simulink model "case14"  (R2018b)
settings: Solver=VariableStepAuto  StartTime=0.0  StopTime=10.0  RelTol=1e-3
(part 2 of 2)

== matlab function case14/MATLAB Function3 ==
  data: y output
function y = fcn()

 u=[0,1,1,1,1,0,1,1,1,1,0,0,1,0,1,0,1,0,1,0,0,1,0,1,1,1,0,1,1,0,0,1,1,0,0,0,1,1,0,0,0,0,1,1,0,0,1,0,1,1,1,0,0,1,1,1,1,0,0,0,0,1,1,1,1,1,0,0,0,1,0,1,1,1,1,1,0,0,0,0,0,1,0,1,1,1,1,0,0,0,0,0,1,1,0,1,1,0,1,0,1,1,0,0,0,0,1,1,1,0,1,1,1,1,0,0,0,0,0,0,0,1,1,0,1,0,1,1,1,1,1,0,0,0,0,0,0,0,1,1,0,0,1,1,1,1,1,1,1,0,1,1,0,0,0,0,0,0,0,1,0,1,1,1,0,1,1,0,1,1,1,0,1,1,0,1,0,0,0,0,0,1,0,1,1,0,1,1,0,1,1,0,1,1,0,1,1,0,0,1,1,0,1,0,0,1,0,1,0,1,0,0,1,1,1,0,1,1,0,1,1,1,1,0,1,1,1,1,0,1,0,0,0,1,0,1,0,0,0,1,0,0,1,1,1,0,0,1,1,1,0,1,1,0,1,1,1,1,1,1,1,0,0,1,0,0,0,0,0,1,0,0,0,0,0,0,1,0,1,1,0,0,0,1,1,1,1,0,1,1,1,0,1,0,1,1,1,0,0,0,1,1,1,1,0,0,0,1,0,0,0,1,0,0,0,0,0,1,1,1,0,1,1,1,1,0,1,0,0,0,1,0,1,1,0,1,1,1,1,1,1,0,0,1,1,0,1,0,0,0,1,0,0,0,0,0,0,0,0,1,0,1,1,1,0,0,1,1,1,0,0,1,1,1,1,0,0,1,1,0,1,1,0,0,1,1,1,1,0,0,1,0,1,0,0,1,0,1,1,0,1,1,0,0,1,0,0,0,0,1,1,0,0,0,1,0,0,1,1,1,0,1,0,0,1,0,1,1,1,1,0,1,1,1,1,1,0,0,1,0,1,1,1,1,1,1,0,0,1,0,1,1,1,1,1,1,0,1,1,0,0,1,0,1,0,0,1,1,0,0,1,0,0,0,0,0,0,1,1,1,0,0,0,1,1,1,1,1,1,1,0,0,0,1,1,1,1,1,1,1,0,0,1,1,1,0,0,1,1,1,1,1,1,0,1,1,1,1,1,1,1,1,0,1,0,1,1,0,0,1,0,0,0,1,0,0,0,0,1,0,0,0,0,1,0,1,0,0,0,1,0,1,1,0,0,0,1,1,1,0,0,1,0,1,0,0,1,1,1,0,1,1,1,0,0,1,1,1,1,1,1,1,0,0,1,1,0,1,1,0,1,0,1,1,0,1,0,1,0,0,1,1,1,0,1,0,1,0,0,0,0,1,0,1,1,1,0,1,0,0,0,1,1,0,0,1,0,1,0,0,0,0,0,0,1,0,1,0,1,1,0,0,1,1,1,0,1,1,1,1,0,1,1,1,0,1,0,1,0,1,1,0,0,1,1,1,1,0,0,0,1,0,1,1,1,1,1,0,1,0,1,1,0,1,0,1,1,1,1,0,0,0,1,0,0,0,0,1,0,1,1,0,0,0,0,1,0,1,0,1,0,0,0,1,0,0,0,1,1,1,0,0,1,0,1,0,1,1,0,1,0,0,1,0,1,0,1,1,0,0,0,1,1,0,1,1,1,1,1,1,0,0,0,1,1,0,1,0,0,0,1,1,1,0,0,1,0,1,1,1,1,1,1,0,1,1,0,1,0,1,1,0,0,0,1,1,0,0,0,1,1,1,0,0,1,0,1,0,0,1,1,0,1,0,0,0,0,1,1,0,0,1,0,0,0,0,0,0,1,0,1,0,0,1,0,0,0,1,1,1,0,0,0,0,1,1,1,1,1,1,0,1,1,0,0,0,0,1,1,1,0,1,1,0,1,1,1,1,1,1,0,0,1,0,1,0,1,1,1,1,1,1,0,0,0,0,1,1,0,0,1,0,1,1,1,1,1,1,1,1,1,0,0,1,0,1,1,0,0,0,1,0,1,1,1,0,1,0,1,1,1,1,0,0,1,0,1,0,0,0,0,1,1,0,0,1,1,0,0,1,0,0,1,1,1,0,0,0,0,0,1,0,0,0,0,0,0,1,0,0,0,1,0,0,1,1,1,1,1,0,0,1,0,1,0,0,1,0,1,1,1,0,1,1,1,0,1,1,1,1,0,0,0,0,0,1,1,0,1,1,1,0,1,0,1,0,1,0,1,1,0,1,0,1,1,1,1,0,1,0,0,1,0,1,1,1,1,1,1,0,1,0,1,0,1,0,0,1,1,1,1,1,1,0,1,0,1,0,1,1,1,0,1,0,0,0,1,0,0,1,1,1,1,0,0,1,0,1,1,0,0,0,0,1,0,0,1,1,0,0,0,0,0,0,0,1,1,1,0,0,0,0,0,1,0,0,1,0,0,1,1,0,0,0,0,0,0,0,1,0,0,1,1,0,1,0,0,0,0,0,0,0,1,1,1,1,1,0,0,1,0,1,1,1,0,0,1,1,0,0,0,1,1,1,1,0,1,0,0,1,1,1,1,1,1,0,0,1,0,0,1,0,1,0,1,1,1,1,1,0,1,1,1,1,0,0,0,0,1,0,1,0,0,0,1,0,1,0,0,0,1,0,0,1,1,1,1,0,0,1,1,1,0,1,1,0,0,0,0,1,1,0,1,1,1,1,0,0,1,0,0,1,1,0,0,0,0,0,0,1,0,0,1,1,0,1,1,1,1,1,1,1,0,0,1,0,0,1,0,0,0,0,1,0,1,0,0,0,0,1,1,1,0,0,1,0,0,1,0,0,0,1,0,1,0,1,0,1,1,0,0,0,1,1,0,0,1,0,1,1,0,1,0,0,1,0,1,1,1,0,0,0,1,1,1,0,1,0,1,1,0,0,1,0,1,1,1,1,0,1,1,0,0,0,1,0,0,0,1,0,1,0,0,1,0,1,1,0,1,1,1,0,1,1,0,1,0,0,0,1,1,0,0,1,1,0,1,0,1,0,1,1,1,1,0,1,1,0,0,1,1,1,1,1,0,1,1,1,0,1,1,1,1,1,1,1,1,0,0,0,0,0,0,1,1,1,0,0,0,1,0,0,0,1,1,0,0,0,1,1,1,1,0,1,0,1,0,0,0,1,1,0,0,0,1,0,0,1,1,0,0,0,0,1,0,0,1,1,0,0,0,1,0,0,1,1,1,1,1,0,0,1,0,0,1,0,0,1,1,1,0,1,1,1,1,1,0,0,1,1,0,1,0,1,1,1,0,1,1,0,0,1,1,0,1,0,0,0,0,1,0,1,1,0,1,1,0,1,1,1,1,1,1,0,1,1,1,1,1,0,0,1,0,0,0,0,1,1,1,1,0,0,1,1,0,0,0,0,0,1,1,1,1,1,1,1,0,1,0,0,1,1,0,1,1,0,1,0,1,0,1,0,1,1,1,1,0,1,1,0,1,1,0,1,1,0,0,1,1,0,1,0,0,1,0,1,0,1,1,1,1,1,0,0,0,1,0,0,1,0,1,0,1,1,0,0,0,1,1,1,0,1,1,0,0,0,0,1,1,1,1,0,0,1,1,0,0,0,0,1,0,0,0,0,1,0,1,0,0,0,0,0,1,0,0,1,0,0,0,1,0,1,0,1,0,1,1,0,0,1,1,0,0,1,0,1,1,1,0,1,0,0,0,1,1,1,1,1,1,0,0,0,0,1,0,0,0,0,1,0,1,1,1,1,1,0,1,0,1,1,0,1,1,1,1,0,0,0,0,1,0,1,0,0,1,0,1,1,1,1,0,1,1,1,1,1,0,0,1,1,1,1,1,1,1,0,1,0,1,0,0,0,0,0,1,1,0,1,1,1,0,1,1,1,1,1,1,1,1,0,1,0,1,1,0,1,0,1,0,0,0,1,1,1,1,1,0,1,0,0,1,1,0,0,1,1,1,0,1,0,1,0,1,0,1,1,1,0,1,1,1,1,0,0,0,1,1,1,0,1,1,1,1,0,0,0,0,0,0,1,1,0,0,1,1,0,1,0,1,0,0,1,1,1,0,0,1,0,1,0,1,0,1,0,0,1,0,0,1,0,0,0,1,1,0,0,0,1,0,1,0,1,1,1,1,1,0,1,0,1,1,1,1,1,0,0,0,0,1,0,0,0,0,1,1,0,1,1,1,0,0,1,0,1,0,1,0,1,0,1,1,1,0,1,0,0,0,0,0,0,0,1,0,0,1,1,0,0,0,0,0,1,1,0,0,0,0,1,1,1,1,0,1,0,1,1,1,1,0,0,0,0,1,0,0,0,1,1,0,1,0,1,1,1,0,0,1,1,1,0,1,1,0,1,1,1,1,1,1,1,0,0,1,1,1,1,1,1,1,1,0,1,0,0,0,1,0,0,0,1,1,1,1,0,0,0,1,1,1,0,1,1,0,0,1,0,0,1,1,1,0,0,1,1,0,1,1,0,1,0,0,0,1,0,0,0,1,0,1,0,1,1,1,0,0,1,1,1,0,1,0,0,1,1,0,1,1,0,1,0,1,0,1,0,1,1,1,0,0,1,1,1,0,1,1,0,0,0,1,1,0,0,0,0,1,1,1,0,1,0,1,1,1,0,1,1,0,0,1,0,0,1,1,0,0,1,1,0,1,0,1,1,0,0,1,0,0,0,0,0,0,1,1,0,0,0,0,1,1,1,1,1,1,0,1,0,0,1,0,0,1,0,0,1,1,1,1,0,0,0,0,1,0,0,0,1,1,1,0,1,0,0,1,0,1,0,0,1,0,1,0,1,0,1,0,0,0,0,0,1,1,1,1,1,1,0,0,1,0,0,0,1,0,0,0,0,1,1,0,0,0,1,1,0,0,0,0,1,1,0,1,1,0,0,0,1,0,1,0,0,0,0,0,0,0,1,1,0,0,0,0,1,1,1,1,0,0,1,1,1,0,1,0,0,0,0,0,0,0,1,0,0,0,1,1,0,1,1,1,0,1,0,1,1,0,1,0,1,1,0,0,1,1,0,1,1,1,1,0,0,0,0,1,0,1,0,0,1,0,1,0,1,1,1,1,0,1,0,1,0,0,0,1,0,0,0,0,0,1,1,1,1,1,1,1,0,1,0,1,0,0,1,0,0,1,1,0,1,0,0,1,1,0,0,1,0,0,1,1,1,1,0,1,1,1,0,1,0,0,0,1,1,1,1,1,1,1,1,0,1,0,1,0,1,0,0,1,1,0,0,1,0,0,0,0,1,0,0,1,0,0,1,1,0,0,1,0,1,0,1,1,0,0,0,0,1,1,1,1,0,1,1,1,1,0,1,0,1,1,0,1,0,1,1,0,0,1,0,1,1,0,0,0,0,0,0,0,1,1,0,1,1,0,0,1,1,1,0,1,0,1,0,0,0,0,0,1,1,0,1,0,1,1,1,1,0,0,0,0,0,0,0,0,1,0,0,0,1,1,0,0,1,0,0,1,0,1,0,0,0,1,0,1,1,1,1,1,0,1,0,1,1,1,0,0,0,0,1,1,1,0,0,0,1,1,0,0,1,0,0,0,1,0,1,1,0,0,1,1,1,0,0,0,0,0,0,0,0,1,0,1,0,1,1,0,1,0,0,1,0,0,1,0,1,1,0,0,1,0,0,0,0,1,1,0,1,1,1,0,0,1,1,0,1,1,0,1,0,0,1,0,1,0,1,1,0,1,1,0,0,0,1,1,1,0,0,1,0,1,0,0,1,1,0,0,1,0,0,1,1,0,1,1,1,1,0,1,1,0,1,0,1,0,0,1,0,1,0,1,0,0,0,1,0,0,0,1,1,1,1,0,1,0,1,1,0,0,1,1,1,1,1,1,1,1,0,0,0,1,0,1,0,0,1,0,0,0,1,1,0,0,1,0,0,0,1,1,0,0,1,1,0,0,0,0,0,1,0,0,1,1,1,1,0,0,1,1,0,1,0,1,1,0,1,1,0,1,1,0,1,1,1,0,0,0,1,0,1,1,1,1,0,0,1,0,1,1,1,1,1,0,0,1,1,0,1,1,0,0,0,1,1,1,0,1,1,1,0,0,1,1,1,1,0,0,0,0,0,1,1,1,0,1,0,1,0,1,1,0,0,1,0,1,1,1,1,0,0,1,0,1,1,1,1,1,0,1,1,1,0,1,0,1,1,0,0,0,0,0,0,0,0,0,1,0,1,1,0,1,0,1,0,0,1,0,1,0,1,1,1,0,0,0,1,0,0,1,1,1,1,0,0,0,0,0,1,1,0,1,1,1,0,1,1,0,0,1,1,0,1,1,0,0,1,0,0,0,0,1,0,1,0,0,0,0,1,0,0,1,0,0,1,0,0,1,0,1,0,0,1,0,1,0,0,0,1,1,0,0,0,0,0,1,1,1,0,0,1,0,0,0,0,1,1,0,1,0,0,1,0,1,1,1,0,1,0,1,0,0,1,0,0,1,1,0,0,0,1,1,1,0,0,0,0,1,0,1,1,1,1,0,0,1,1,1,0,1,1,1,0,1,0,0,0,0,1,1,0,1,1,0,1,1,0,0,0,1,1,1,0,1,1,0,1,1,0,1,1,0,1,0,0,1,0,1,1,0,1,1,0,0,0,0,1,0,1,0,0,1,0,0,0,1,1,1,0,0,1,1,1,1,0,0,0,1,0,1,0,1,0,1,1,1,1,1,0,0,1,1,1,1,0,1,0,1,1,1,1,0,0,0,1,1,1,0,0,0,0,0,1,0,0,1,0,1,1,1,1,1,1,0,0,0,0,1,1,1,0,0,0,0,1,0,1,0,1,0,0,1,1,1,1,1,1,1,1,1,1,1,0,1,1,0,1,1,0,0,0,0,0,1,0,1,0,0,0,1,0,1,0,0,1,1,0,0,0,1,0,0,0,1,1,0,0,1,0,1,1,1,0,1,1,0,1,1,1,1,0,0,0,1,1,1,0,0,0,1,0,1,0,0,0,0,0,1,1,1,1,0,0,1,1,0,0,0,0,1,0,0,0,1,1,0,1,1,0,1,1,1,1,1,0,1,0,0,1,0,1,0,1,1,0,0,1,0,1,1,1,0,0,1,1,0,0,1,1,1,0,0,1,0,1,0,1,1,1,1,0,1,0,0,0,1,0,1,1,0,1,0,1,0,1,0,0,1,0,1,1,1,1,1,1,0,0,0,1,1,0,1,1,0,0,0,0,0,0,0,0,1,0,0,1,0,1,0,1,0,1,1,1,0,1,1,1,0,0,0,0,0,1,0,1,0,0,1,0,0,1,0,1,1,0,0,1,0,0,0,0,1,1,0,0,1,0,0,0,1,1,0,1,1,0,1,0,0,0,0,0,1,0,1,0,0,0,0,0,1,0,0,1,1,0,1,0,1,0,0,0,1,0,0,1,0,1,0,1,1,0,1,0,1,0,1,0,1,0,1,1,0,1,0,0,0,0,0,0,1,0,0,1,0,1,0,0,0,1,1,0,0,1,1,0,1,1,1,1,1,1,1,1,0,0,1,1,0,1,1,1,1,0,0,1,1,1,1,0,1,0,1,1,0,0,0,1,0,0,0,0,1,0,0,1,1,0,0,1,0,0,1,0,0,0,1,1,1,1,1,0,1,1,0,1,1,0,1,0,1,0,1,1,1,0,0,1,0,0,1,1,1,0,1,0,1,1,1,0,1,0,1,1,0,0,1,0,0,0,1,0,0,0,0,1,0,1,0,1,0,0,1,1,1,1,0,0,1,1,1,1,1,0,0,0,1,1,1,1,1,0,1,1,1,1,1,1,1,1,1,0,0,1,1,1,0,1,1,0,1,0,0,1,1,0,0,1,1,0,0,0,0,0,0,0,1,1,1,1,1,0,1,0,1,0,0,0,1,1,0,0,0,0,1,1,1,1,0,0,0,0,1,0,1,0,1,0,0,0,1,0,0,0,1,1,0,0,1,0,0,1,1,1,1,0,1,0,0,1,1,1,1,1,1,0,1,1,0,0,0,1,0,1,1,0,1,1,1,1,0,1,1,1,1,1,1,1,1,0,0,1,0,0,0,0,0,1,0,0,0,1,1,0,1,1,0,0,0,1,1,0,1,1,0,0,1,0,0,1,1,0,0,1,0,0,1,1,1,1,1,0,0,1,0,1,1,1,0,0,1,1,0,0,1,1,0,0,1,0,0,1,0,1,1,0,0,1,0,1,1,1,0,1,0,1,0,0,1,1,1,0,0,1,0,1,0,1,1,1,0,1,1,0,0,1,1,0,1,0,1,1,1,0,1,0,0,1,1,1,0,1,1,0,1,1,1,1,1,0,1,0,0,1,0,1,0,1,0,1,1,0,0,1,0,1,0,0,0,0,1,1,1,0,0,1,1,1,1,0,1,1,0,1,0,0,1,1,0,0,1,1,0,1,1,1,0,1,1,1,0,0,1,0,1,0,1,1,0,0,1,0,0,0,0,1,0,0,0,1,0,0,0,1,0,0,1,1,0,1,0,0,1,1,1,1,0,1,0,1,0,1,0,1,0,1,1,1,1,0,0,0,0,1,0,0,0,0,1,1,1,1,1,1,1,0,0,0,1,0,0,0,1,0,1,0,1,1,1,0,0,1,0,1,0,0,0,1,1,0,0,1,0,0,0,1,1,0,1,0,0,1,1,0,0,1,1,1,1,1,1,0,0,1,0,0,1,0,1,0,1,0,0,1,1,0,1,1,0,0,1,1,1,1,1,0,1,0,1,0,1,1,1,1,0,0,0,0,1,1,1,1,1,0,1,0,1,0,1,1,1,0,1,1,0,1,1,0,0,0,0,1,0,0,1,1,0,0,0,1,0,1,1,0,1,1,1,0,1,0,0,0,0,0,0,0,1,1,1,0,1,0,0,1,1,0,1,0,0,1,0,1,1,1,0,0,0,1,1,1,1,1,1,1,0,0,0,0,1,1,1,1,0,0,1,0,1,0,0,0,1,1,0,1,0,1,0,1,1,1,0,0,0,1,0,0,1,1,0,1,1,1,0,0,1,0,1,0,1,1,0,1,0,1,1,0,1,0,1,0,0,0,1,1,0,0,0,0,1,1,1,0,0,0,1,0,1,1,0,0,1,1,0,1,1,0,0,0,1,1,0,1,1,1,1,0,1,1,0,1,0,1,1,0,1,0,1,1,0,1,1,0,1,1,0,0,0,1,0,1,1,1,1,0,0,1,0,0,0,1,0,1,1,1,1,1,1,1,0,0,1,0,0,1,1,0,1,0,1,1,0,0,1,0,1,0,0,0,0,0,1,0,0,0,0,0,1,0,1,0,0,0,0,1,1,1,1,0,0,1,1,0,0,1,1,0,1,1,0,1,0,1,1,1,0,0,0,0,0,0,0,1,0,1,0,1,1,1,1,0,0,0,0,0,0,0,0,0,1,0,1,1,1,0,1,1,1,1,1,0,0,1,1,1,0,1,0,1,1,1,0,0,0,0,1,0,0,1,0,1,1,1,1,0,1,0,1,0,0,0,0,1,0,0,0,1,1,0,0,0,0,0,0,0,1,1,1,1,1,0,0,0,1,0,0,0,0,0,1,1,0,0,1,1,0,0,0,1,1,0,0,1,1,1,0,1,1,0,0,0,1,0,0,0,0,1,0,1,0,0,0,0,1,0,1,1,1,1,1,1,1,0,1,1,0,1,0,0,1,1,0,0,0,1,0,1,1,1,0,1,0,0,0,0,0,1,1,0,1,0,0,1,0,0,0,1,1,1,1,0,0,1,0,0,0,0,0,1,1,0,1,0,0,1,1,0,1,0,0,1,0,0,0,0,1,0,0,1,1,1,0,1,0,0,0,0,0,1,0,0,0,0,0,1,1,0,1,0,0,1,0,1,0,1,0,1,1,0,1,1,1,0,1,0,0,0,0,1,1,0,1,0,1,0,0,1,1,1,0,0,0,0,0,0,0,0,0,1,0,0,0,1,1,1,0,1,0,1,0,0,1,0,1,0,0,1,1,1,1,1,1,0,0,0,1,1,0,1,1,0,1,1,0,1,1,0,0,1,1,0,1,1,0,0,0,0,1,0,1,1,0,0,1,1,1,1,1,0,1,1,0,0,0,0,0,1,0,1,1,1,0,1,1,0,0,1,0,1,1,0,0,0,1,0,0,1,1,1,1,1,1,1,1,1,0,0,1,0,0,1,1,1,0,1,0,0,0,1,1,0,0,1,0,1,0,0,0,1,0,0,1,1,1,1,1,0,1,1,1,1,1,0,1,1,0,1,1,0,0,1,1,1,0,1,0,1,1,0,0,1,0,0,1,1,1,1,0,1,1,1,0,0,0,1,1,1,1,0,0,0,0,1,1,0,0,0,0,1,1,1,1,0,1,0,1,1,0,0,1,0,1,0,1,1,0,0,1,0,0,1,0,1,0,1,1,1,1,1,1,0,1,0,1,0,1,0,1,1,1,1,0,0,1,1,0,1,1,1,0,0,1,0,0,0,0,1,1,0,1,1,0,0,0,1,1,1,0,0,0,1,0,0,0,1,1,0,0,0,0,1,1,0,0,1,0,1,1,1,1,1,0,1,0,1,1,1,0,1,1,1,0,0,1,0,1,1,0,0,0,1,0,0,0,0,1,0,1,1,1,0,1,0,0,0,1,0,1,0,1,1,1,0,0,1,1,1,0,0,1,0,1,0,0,0,1,1,0,0,1,1,1,1,0,0,0,0,1,1,0,0,1,1,1,0,0,1,0,0,0,0,0,0,0,1,0,1,0,1,1,1,1,1,0,0,1,0,1,0,0,0,0,1,1,1,1,0,1,0,0,0,1,1,0,0,1,0,0,0,0,1,0,1,0,1,0,0,1,0,1,1,0,0,1,0,0,1,1,1,1,0,1,0,1,0,0,0,0,0,0,1,0,0,0,1,0,1,0,0,0,0,1,0,0,0,0,1,0,0,1,1,1,1,0,1,0,0,1,0,0,0,0,1,1,0,0,0,1,1,0,0,0,0,0,1,1,0,0,0,1,1,1,0,1,1,1,0,1,0,0,1,1,1,0,0,1,0,1,0,1,0,0,1,0,1,0,0,0,1,1,1,1,1,1,1,0,1,0,0,0,0,1,1,1,1,0,0,0,0,1,1,0,1,0,1,0,0,1,1,0,1,1,0,1,0,0,1,0,1,1,1,1,0,1,1,0,1,0,0,0,1,0,0,0,1,0,1,0,1,0,0,1,0,0,0,1,0,0,0,1,0,1,0,0,0,1,1,0,1,0,0,1,0,0,1,0,0,1,1,0,0,1,0,1,0,0,0,0,1,1,1,0,1,0,0,0,1,0,1,1,1,1,0,0,1,1,0,1,1,1,0,0,1,0,1,1,0,1,1,0,0,1,1,1,0,0,0,1,1,0,0,0,0,1,0,0,0,1,1,0,0,1,0,1,1,0,1,1,0,1,1,0,1,0,0,0,0,1,1,1,1,1,0,0,1,0,0,1,1,0,1,1,0,0,0,0,0,1,1,1,1,0,1,0,0,1,0,0,1,0,0,1,0,1,1,0,0,1,1,1,0,1,1,1,1,0,0,1,1,1,0,0,0,1,1,0,0,1,0,0,1,0,1,1,0,0,0,1,0,0,1,1,0,0,0,0,1,0,1,1,1,0,1,0,0,0,1,1,1,1,0,1,0,1,1,0,0,1,1,0,1,1,0,1,1,0,1,0,0,1,1,1,0,1,0,1,1,1,0,1,1,1,0,1,1,0,1,0,1,0,1,1,1,0,1,1,1,0,1,0,0,1,0,0,0,0,1,0,1,1,0,1,0,0,1,0,0,1,1,0,1,0,1,0,0,1,1,1,1,0,0,0,0,1,1,1,1,0,1,0,0,0,0,0,0,0,1,1,1,0,1,0,1,1,0,1,0,1,0,1,1,0,0,0,1,1,0,1,0,0,0,1,0,0,0,1,1,1,0,0,1,1,1,1,1,0,0,1,1,1,0,0,1,1,1,1,0,1,1,0,1,0,0,0,0,1,1,0,1,1,1,1,0,1,1,1,1,0,1,0,1,1,1,0,1,1,1,1,1,1,0,1,0,1,0,0,0,0,1,1,0,1,1,0,0,1,0,1,1,0,1,0,1,0,1,1,1,1,0,1,1,0,0,1,1,1,0,1,0,0,0,0,1,1,1,1,0,1,0,1,1,0,0,0,0,0,1,0,1,0,1,1,1,1,1,1,1,0,1,1,0,0,0,1,1,0,0,1,1,1,1,0,0,0,0,1,1,0,0,1,1,1,0,1,0,1,1,0,0,0,1,1,0,0,0,1,0,1,0,1,1,1,0,1,0,0,0,1,0,1,1,1,1,0,1,1,1,0,0,1,0,1,1,0,0,0,1,0,0,0,1,0,1,0,0,0,0,0,1,0,1,1,0,0,1,1,1,1,0,0,1,1,1,0,1,1,1,0,0,0,1,1,1,0,0,1,0,0,1,1,1,1,0,1,1,0,0,0,1,0,0,1,1,0,0,0,0,1,0,1,0,1,0,1,0,0,0,0,0,0,1,0,1,0,1,1,0,1,1,0,0,1,0,1,0,1,1,0,0,1,0,1,0,0,0,0,1,1,1,1,0,0,1,1,1,1,0,0,0,0,1,1,1,0,0,0,1,0,0,0,0,1,1,0,1,1,0,0,1,0,1,0,0,0,1,1,0,0,1,0,0,1,0,0,0,0,0,1,0,0,0,0,0,1,1,0,1,1,1,0,1,0,1,1,0,0,1,1,1,0,1,0,0,0,1,1,0,1,1,0,0,0,0,0,0,0,0,0,1,1,0,1,1,1,0,0,1,0,1,1,0,0,1,0,0,0,1,0,1,1,1,1,1,0,0,1,0,0,0,0,0,1,1,0,0,1,0,1,1,1,1,0,0,1,0,0,1,1,0,0,1,0,0,1,0,0,1,0,0,1,1,1,0,0,0,0,0,0,1,1,0,1,0,1,1,0,1,0,1,0,0,0,1,1,1,0,1,1,1,1,1,1,1,1,1,0,0,0,1,1,0,1,0,1,0,0,1,1,1,1,0,1,0,0,0,1,0,0,1,0,1,0,1,0,1,1,0,1,0,0,1,1,1,1,1,0,1,1,1,1,1,0,1,0,0,0,1,1,0,1,1,1,1,0,1,1,0,1,0,0,1,1,0,1,0,0,1,1,1,1,1,0,1,1,0,0,0,0,1,1,1,0,1,1,0,1,0,0,1,1,1,1,1,0,1,0,0,0,1,0,1,1,1,0,0,1,1,0,1,0,0,1,0,0,0,0,0,0,0,1,0,1,1,1,1,0,1,0,1,1,1,1,0,1,1,1,0,0,1,0,0,0,1,1,0,0,1,1,1,0,0,1,1,0,0,1,1,1,1,1,0,1,1,1,0,0,0,0,0,1,1,1,1,1,1,1,0,0,1,1,1,0,1,1,1,1,0,1,0,1,0,0,0,0,1,0,1,1,0,1,1,1,1,0,0,0,1,0,1,0,0,0,1,1,0,0,0,0,0,1,0,0,0,1,0,1,1,1,1,1,1,1,1,1,0,0,0,0,1,0,1,0,1,1,1,1,1,1,1,0,0,0,1,0,1,0,0,1,0,0,1,1,0,0,1,1,0,0,0,0,1,1,1,1,0,1,0,1,1,1,1,1,0,1,1,1,1,1,0,1,0,1,1,0,0,1,0,1,0,0,1,1,0,1,1,0,0,0,0,0,0,0,1,0,1,1,1,0,1,1,0,0,0,0,1,0,1,1,1,0,0,1,0,0,1,0,0,1,0,1,0,0,1,0,1,0,0,1,0,0,0,0,1,0,0,1,1,1,0,0,1,0,0,1,1,0,0,1,0,1,1,1,0,0,0,1,1,1,1,0,0,1,1,1,0,1,0,1,0,0,1,0,1,0,0,1,0,1,0,1,1,0,0,0,1,0,0,1,1,0,1,1,1,0,0,0,1,0,1,0,1,0,0,1,1,1,0,1,0,1,1,0,0,0,0,1,1,1,1,0,0,0,0,0,0,0,1,1,1,0,0,0,1,0,1,1,0,1,0,0,1,1,0,1,0,0,0,1,1,1,1,1,1,1,0,1,0,0,0,1,0,0,1,0,1,1,1,0,0,1,1,0,1,1,1,1,0,0,1,0,0,1,0,0,0,1,0,1,0,1,0,0,0,0,0,1,1,1,1,0,0,0,0,1,0,1,0,1,0,0,0,0,0,1,1,0,0,1,0,0,1,1,0,1,0,1,0,1,1,0,1,1,0,0,0,0,0,0,1,1,0,0,1,1,0,1,0,0,1,1,1,0,1,1,0,0,1,1,1,0,1,0,1,1,0,0,0,1,0,1,0,1,1,1,0,1,1,1,0,0,0,0,0,0,0,1,1,1,1,0,1,1,1,1,0,0,0,0,1,0,1,0,1,0,1,0,1,0,0,0,0,1,1,0,1,0,0,1,1,0,1,1,1,0,1,1,1,0,1,1,1,1,0,1,1,0,0,1,0,1,0,1,1,0,0,0,1,0,0,0,1,0,0,1,1,0,0,1,1,0,1,0,0,1,0,0,0,0,1,1,0,0,0,1,1,1,1,0,1,0,1,1,0,0,1,0,1,0,1,0,1,1,0,1,0,0,0,0,0,1,0,0,1,0,0,0,1,1,0,1,0,0,0,1,0,1,0,0,1,1,0,0,1,0,0,0,1,0,1,0,1,1,0,0,0,1,1,0,1,0,1,0,0,0,1,0,1,1,0,0,1,0,1,1,0,1,1,0,0,1,1,0,0,1,1,0,0,0,1,0,1,1,0,0,0,0,0,1,1,0,1,1,0,0,1,1,0,1,1,0,0,1,0,0,1,1,1,0,0,1,0,0,1,1,1,0,1,1,1,1,1,0,1,1,0,0,0,0,0,0,0,0,1,0,0,0,0,1,0,0,1,0,1,1,1,0,0,1,0,0,0,0,0,0,1,1,0,1,0,0,0,0,1,1,0,1,1,0,0,1,1,1,0,1,1,1,0,1,0,1,0,1,1,1,1,0,0,0,0,1,1,1,1,0,0,1,1,1,0,1,0,1,0,0,0,0,0,1,1,1,1,1,1,1,0,0,1,1,0,0,1,1,0,1,0,0,1,0,0,0,1,1,0,0,0,0,0,0,0,0,0,1,0,0,0,0,0,1,1,1,0,0,0,0,0,1,1,0,0,0,0,1,1,0,1,0,1,0,1,1,1,1,0,1,1,1,0,1,1,0,0,1,0,1,0,0,0,1,0,1,0,0,0,1,1,0,1,1,0,0,0,1,0,1,0,1,0,0,1,0,0,1,0,0,0,0,0,1,1,1,0,1,1,0,1,1,0,0,1,1,0,1,1,1,1,0,1,1,1,0,0,1,0,1,0,0,0,0,1,1,0,0,0,0,1,0,0,1,1,0,0,0,0,0,0,0,0,1,0,0,1,1,0,0,1,1,1,0,1,0,1,1,0,1,1,1,1,1,1,0,1,0,0,1,0,1,0,1,0,1,0,1,0,0,1,0,1,0,1,1,0,1,1,1,0,1,0,1,0,0,1,1,0,1,1,1,1,1,0,1,0,1,1,1,1,1,0,1,0,0,1,0,0,1,1,1,0,1,1,0,0,1,1,1,1,0,1,1,0,0,1,0,1,1,0,1,1,0,1,0,1,1,1,1,1,0,0,0,1,0,0,0,1,0,1,0,1,0,1,1,0,1,1,1,1,1,1,1,1,0,0,1,0,0,1,1,1,0,0,0,0,0,0,1,0,1,1,0,1,0,1,0,1,0,0,1,0,1,1,1,0,1,0,0,0,0,1,0,1,0,1,1,0,0,0,1,1,0,0,1,1,0,0,0,1,0,1,1,0,0,1,0,1,0,1,1,0,1,0,0,0,0,0,1,0,0,1,0,0,1,1,1,0,1,1,1,1,0,0,1,1,0,0,0,0,1,1,1,1,1,0,1,0,1,1,1,0,0,0,1,1,1,0,0,0,0,1,0,0,1,0,0,0,1,0,1,1,0,0,1,1,1,0,1,1,1,0,0,1,1,0,1,0,1,1,1,0,1,0,1,1,1,1,1,0,0,1,0,0,1,0,0,0,0,0,0,0,0,0,0,0,1,1,0,1,0,1,0,1,1,1,1,0,0,0,1,1,1,1,0,0,0,0,0,0,1,0,1,1,0,1,1,1,1,1,0,0,0,1,1,1,0,0,0,0,1,0,1,0,0,0,0,1,1,0,0,0,0,0,1,0,1,0,1,0,1,1,1,0,0,0,0,1,1,0,0,0,1,1,1,0,1,1,0,1,0,1,1,1,1,0,0,1,0,0,1,0,1,1,0,1,0,0,1,0,0,1,0,0,1,0,0,0,1,1,1,0,0,1,0,0,1,0,0,1,1,1,1,0,1,0,0,0,1,0,0,0,1,1,0,0,0,0,1,0,1,1,1,1,0,0,0,1,1,1,0,0,1,1,0,1,1,0,1,0,1,0,0,0,1,0,1,1,0,1,0,0,1,1,1,1,0,1,1,0,0,0,1,1,1,1,1,0,0,1,1,1,0,1,0,1,1,0,1,0,1,1,0,1,1,0,1,1,0,1,1,1,1,0,1,0,1,1,1,1,0,1,1,0,0,1,0,0,1,1,0,0,1,0,0,0,1,0,0,1,1,1,1,1,0,0,0,0,1,1,0,1,1,1,0,0,0,1,0,1,0,1,1,0,1,0,1,0,0,1,0,1,1,1,1,1,1,1,1,1,0,0,1,0,1,0,0,0,1,0,0,0,0,0,1,0,1,1,0,0,0,0,1,0,1,1,0,0,1,0,1,0,1,0,0,0,1,1,1,1,1,0,0,0,0,1,1,0,0,0,1,0,0,0,1,1,1,0,0,1,0,0,1,1,0,0,0,0,0,1,0,1,1,0,0,0,0,1,0,1,1,1,0,0,0,1,0,0,1,0,0,1,0,0,1,0,1,0,0,1,1,0,0,0,0,1,1,0,1,1,1,1,1,0,0,1,1,0,0,1,1,1,0,1,1,0,0,1,1,1,0,1,1,0,1,0,1,1,1,0,0,0,0,0,0,0,0,1,1,0,0,1,0,1,0,0,0,0,1,1,1,0,1,1,1,0,1,0,1,0,1,1,0,1,0,1,0,0,1,0,0,0,0,1,0,0,1,1,0,1,1,0,0,1,1,0,1,0,1,1,0,0,0,1,1,1,0,0,1,0,0,1,0,1,0,1,1,0,1,0,0,1,0,0,1,1,0,0,0,1,0,0,1,1,1,1,0,1,1,0,0,1,0,1,1,0,1,1,0,1,0,0,1,0,1,0,1,1,1,1,1,1,1,1,0,0,0,1,1,0,0,1,0,1,1,1,0,1,1,0,0,1,1,1,0,0,0,1,1,1,1,0,0,0,1,0,1,0,0,0,0,0,1,0,1,1,1,0,1,0,1,1,0,1,1,0,0,1,1,1,0,1,1,1,1,1,1,1,1,0,0,0,0,1,0,1,0,0,1,1,1,1,1,0,1,0,1,0,0,0,1,1,0,0,1,0,0,1,1,1,1,1,1,1,0,0,1,0,1,1,0,0,1,0,1,0,0,1,0,1,0,0,0,0,1,0,0,0,0,1,1,1,1,0,0,1,0,1,0,1,1,0,0,1,1,0,1,1,0,1,1,1,1,0,1,1,0,0,1,1,0,1,0,1,0,1,0,0,0,0,0,0,0,0,1,1,1,0,1,0,0,0,1,0,0,0,0,1,1,0,1,1,0,0,1,1,0,1,0,0,1,1,0,1,1,0,1,0,1,0,0,0,0,0,0,0,1,1,1,1,1,0,1,1,1,0,1,0,1,0,0,0,0,1,0,1,0,1,1,0,1,0,1,1,1,1,0,0,0,0,1,0,0,1,1,0,0,1,0,1,0,0,1,0,1,0,0,0,1,0,0,1,1,1,0,1,1,1,1,1,1,1,0,1,0,0,0,1,1,0,0,0,0,1,1,1,1,0,0,1,1,1,1,1,1,1,0,1,0,1,1,1,0,0,1,0,0,1,1,1,1,0,0,1,1,1,0,0,1,1,1,1,0,1,1,1,0,1,1,0,0,0,0,0,0,1,1,1,1,1,0,1,0,1,0,1,0,1,1,0,1,0,1,1,0,1,0,0,0,1,1,1,0,1,1,1,1,0,0,0,0,1,1,0,1,1,0,1,1,0,1,0,0,0,0,0,0,1,1,1,1,0,0,1,1,1,1,1,1,0,1,1,0,0,1,0,1,0,0,1,1,0,0,1,1,0,1,1,0,0,1,0,0,0,1,0,1,0,0,0,1,1,1,1,0,0,1,1,1,0,0,1,0,0,0,1,1,0,0,0,1,0,1,0,1,0,1,0,0,1,0,0,1,1,0,1,0,0,0,1,1,0,0,0,1,0,1,0,1,1,1,0,1,1,1,0,1,0,0,1,0,0,1,1,0,0,0,1,1,0,1,1,0,0,1,0,0,0,1,1,1,0,0,0,0,1,1,1,0,1,1,1,0,1,0,0,0,0,0,0,0,0,1,1,0,0,0,0,0,0,0,1,0,0,1,0,0,0,1,1,0,0,0,1,0,1,0,0,1,1,1,0,1,1,1,1,0,0,0,0,1,0,1,0,0,0,0,1,1,1,1,0,0,1,1,1,1,1,0,0,1,1,0,1,1,1,1,1,1,1,0,1,0,0,0,1,0,1,0,1,0,1,0,1,1,0,0,0,1,0,0,1,1,1,1,0,1,1,1,1,0,0,0,0,0,1,0,1,0,0,0,0,0,1,0,1,0,1,1,1,0,0,1,1,1,0,1,1,0,1,1,0,1,0,1,0,1,0,1,1,0,0,0,1,1,0,1,0,1,0,0,1,1,0,0,1,1,1,1,1,1,0,0,0,0,1,0,0,0,1,1,1,0,0,0,0,1,0,0,0,1,0,1,0,1,0,1,0,0,0,1,1,0,0,1,1,0,1,0,0,0,0,0,1,1,1,0,1,0,1,0,0,1,0,1,0,0,0,0,0,0,0,0,1,0,0,0,1,0,0,1,1,1,1,1,0,1,0,1,0,0,0,0,0,0,0,1,1,0,0,0,0,0,1,0,0,0,0,1,0,1,1,0,1,0,1,1,1,1,0,0,0,0,1,0,0,1,0,1,0,0,0,0,0,1,0,1,1,1,1,0,1,1,1,1,0,0,0,0,0,0,1,1,1,0,1,0,0,0,1,0,1,1,0,0,1,1,0,0,1,0,1,0,1,0,1,1,1,0,1,1,0,1,1,1,1,1,0,1,0,1,1,1,1,0,1,1,1,1,0,0,1,1,0,0,0,0,1,1,1,1,0,0,1,0,0,0,1,1,1,0,0,1,0,1,0,1,1,0,1,1,1,0,0,0,0,0,1,0,1,0,1,1,0,1,0,0,1,1,0,0,1,0,0,1,0,0,1,0,0,0,0,1,0,1,0,1,0,1,0,0,1,0,0,1,1,0,1,0,0,0,0,0,0,0,1,1,1,1,1,0,0,1,1,0,0,0,0,1,1,1,1,0,1,1,0,0,0,0,0,1,0,0,0,0,0,0,1,0,0,1,0,0,1,0,1,1,1,1,0,1,0,0,1,1,0,0,1,0,0,0,1,0,1,0,0,1,1,0,0,0,0,0,1,0,0,0,1,1,0,1,1,0,1,1,0,0,0,0,0,1,1,0,1,1,1,0,0,1,1,0,1,1,1,1,0,0,1,1,0,1,1,1,0,0,1,1,1,0,1,0,1,0,0,0,0,1,1,1,0,0,1,1,1,0,1,1,1,0,0,0,1,1,1,1,1,1,0,0,0,0,0,0,0,0,1,0,0,0,1,0,0,0,0,0,1,1,0,0,1,0,0,0,0,1,0,1,0,1,0,0,1,1,0,0,1,1,1,0,1,0,0,1,0,0,0,1,0,0,1,0,1,1,0,1,0,1,1,1,0,1,1,1,0,0,1,0,0,0,0,1,0,1,1,0,0,1,0,1,0,0,0,1,1,1,0,0,0,1,0,1,1,0,1,0,0,1,0,1,1,0,0,1,1,1,0,0,1,0,1,0,1,0,1,1,1,0,1,1,0,1,1,0,0,0,1,1,1,1,0,1,0,1,1,1,1,0,1,1,0,1,1,0,0,0,0,0,0,0,1,0,0,1,1,0,1,1,1,1,1,1,0,0,1,1,0,1,1,0,0,0,0,1,0,0,1,1,1,1,0,0,1,0,0,0,1,1,0,0,0,0,1,1,0,1,1,1,0,1,0,1,1,1,0,1,0,1,1,1,1,0,0,0,0,1,0,0,0,0,0,1,0,1,0,1,1,0,1,1,0,0,0,0,0,0,1,1,0,1,0,0,0,0,1,1,1,0,0,1,1,0,0,0,1,0,1,1,0,0,0,0,0,1,1,1,1,1,1,1,0,1,0,0,1,1,0,1,1,1,1,1,1,1,0,0,1,1,0,1,1,0,1,1,1,1,1,0,0,0,1,1,1,1,1,1,1,0,0,1,1,0,1,1,1,1,0,0,1,0,1,1,0,0,0,0,1,1,0,1,1,1,0,1,0,0,0,1,0,1,0,1,0,0,0,0,0,0,1,1,0,1,0,1,0,1,0,0,0,0,0,0,1,0,1,1,0,1,0,0,0,0,1,0,1,0,0,1,0,1,0,1,0,1,0,0,0,1,0,0,1,1,1,1,1,0,0,0,0,1,0,0,0,1,0,0,0,1,0,1,1,0,1,0,1,1,0,0,0,0,0,1,1,0,1,1,1,0,1,1,1,1,1,1,0,1,1,1,1,1,0,0,0,1,1,0,1,1,0,0,1,1,0,0,1,1,1,1,0,1,0,1,1,0,0,0,0,1,0,1,0,0,0,1,0,1,1,1,0,0,1,0,1,1,0,0,0,0,0,0,0,0,0,1,0,1,1,0,0,1,1,1,1,0,0,0,0,0,0,1,0,1,0,1,1,0,0,0,0,0,0,1,0,0,1,0,0,0,1,1,1,1,0,0,1,0,0,0,0,0,0,1,1,1,1,0,0,0,1,1,1,0,1,1,0,1,0,1,1,1,1,1,1,0,1,1,0,0,1,1,1,1,0,1,0,0,1,1,0,1,0,1,1,0,0,0,1,1,1,0,0,1,1,1,0,0,1,0,1,0,0,1,0,0,0,0,0,0,1,0,1,1,0,0,0,1,1,1,0,1,0,0,1,1,1,0,0,0,0,0,0,1,0,0,1,1,1,0,0,1,0,1,0,1,1,0,1,0,0,1,0,1,0,1,1,0,0,0,1,1,1,0,1,1,1,0,1,0,1,0,1,1,1,1,0,0,1,0,1,1,1,1,0,1,1,1,0,0,0,0,1,0,1,0,0,1,0,1,0,0,0,0,0,1,0,1,1,1,0,0,0,0,1,1,0,0,1,0,1,0,1,0,0,0,1,0,0,0,0,1,0,0,0,1,1,0,0,1,0,1,0,1,1,1,1,1,1,0,1,0,1,1,0,0,1,1,1,0,1,0,0,0,1,0,1,1,1,1,0,1,0,1,0,0,0,1,1,0,1,0,1,0,0,1,0,1,0,0,1,0,0,1,1,0,0,0,0,0,0,0,1,1,0,0,0,1,0,0,0,1,1,0,1,0,1,1,0,0,0,1,1,1,0,0,1,0,1,1,1,0,1,0,1,1,1,1,0,1,1,1,1,0,1,1,1,0,1,1,0,0,1,0,1,0,0,0,0,0,0,0,0,1,0,0,0,0,0,0,1,1,0,0,0,1,1,0,0,0,0,0,0,0,1,1,1,0,0,0,0,0,0,0,1,1,1,0,0,0,1,1,1,1,1,1,0,1,1,0,0,1,1,0,1,0,1,1,0,0,1,0,0,0,0,0,0,1,0,1,1,0,0,0,0,0,0,1,0,1,1,0,0,0,0,0,1,0,0,0,0,1,0,1,1,0,1,0,0,0,1,1,0,1,1,1,0,0,1,1,1,1,0,1,1,0,0,1,0,0,1,0,1,1,0,1,0,1,1,0,0,0,0,1,1,0,0,1,0,0,1,1,0,0,0,0,1,1,0,0,0,1,1,0,0,0,1,0,1,1,1,1,1,1,1,1,0,1,1,1,0,1,0,0,1,1,0,0,0,0,0,0,1,0,0,1,0,1,1,1,0,1,0,0,0,0,1,0,0,0,1,1,1,1,1,0,1,1,1,0,1,1,1,0,0,0,0,1,1,1,0,0,0,1,0,1,0,0,0,1,0,0,0,0,1,1,1,0,0,1,0,1,1,1,1,1,1,0,1,1,1,1,1,0,1,1,0,0,0,0,0,0,0,1,0,0,1,0,0,0,1,1,0,0,0,1,1,0,1,1,1,0,1,0,1,1,1,0,1,0,0,0,0,1,0,0,0,0,1,0,0,1,0,0,0,1,1,0,1,0,1,0,1,1,0,1,0,0,1,1,0,0,1,0,0,1,0,0,1,0,0,1,0,0,1,0,1,1,1,1,1,0,1,0,0,1,0,0,0,1,0,0,1,0,0,0,1,0,1,1,1,1,1,1,1,0,0,1,0,0,0,0,0,0,0,1,1,0,0,1,1,1,1,1,1,1,0,0,0,0,0,1,0,1,0,0,1,1,1,1,1,1,1,0,0,0,0,1,0,0,0,1,1,1,1,0,0,1,0,1,0,0,1,0,0,1,1,1,1,1,0,0,0,0,1,0,1,1,1,1,1,0,0,0,0,0,1,0,1,1,1,0,0,0,0,0,1,1,1,1,0,0,0,0,1,1,0,0,0,1,0,1,1,0,0,1,1,1,1,0,0,1,1,1,0,0,1,1,0,0,1,0,0,0,1,0,1,1,0,1,0,1,0,1,0,1,1,0,0,0,0,1,0,0,0,0];

 y = u;

== matlab function case14/MATLAB Function4 ==
  data: y output
function y = fcn()
 u=[5111, 5109, 5108, 5106, 5103, 5101, 5100, 5098, 5095, 5094, 5093, 5091, 5090, 5081, 5080, 5069,5068, 5054, 5044, 5027, 5026, 5014, 5004, 4980, 4915, 4909, 4893, 4885, 4832, 4824, 4591, 3706,5092, 4986, 4965, 4920, 4917, 4858, 4847, 4790, 4770, 4318, 4126, 3961, 3790, 4911, 4881, 4827,4795, 4789, 4725, 4675, 4539, 4535, 4458, 4197, 4096, 3484, 3481, 3393, 3175, 2360, 1852];
y = u;

== matlab function case14/MATLAB Function5 ==
  data: y output
function y = fcn()
 u=[412, 161, 1, 303, 207, 4971, 4496, 5, 4557, 485, 253, 4676, 1, 66, 4485, 282,193, 5211, 729, 4848, 982, 5955, 9805, 670, 464, 29, 429, 394, 616, 9457, 4429, 4771,365, 9705, 9489, 4193, 9947, 824, 864, 347, 677, 6544, 6312, 9804, 278, 9461, 444, 4839,4144, 9875, 197, 1156, 4674, 10035, 4504, 5, 9937, 430, 5, 355, 909, 1622, 6284];
y =int32(u);

== matlab function case14/Switch Case Action Subsystem1/For Iterator Subsystem/GetGpsL1C/If Action Subsystem/Subsystem/For Iterator Subsystem1/If Action Subsystem/If Action Subsystem1/MATLAB Function ==
  data: value input; y output; index input
function y = fcn(value,index)

y = value(index);

== matlab function case14/Switch Case Action Subsystem1/For Iterator Subsystem/GetGpsL1C/If Action Subsystem/Subsystem/For Iterator Subsystem/If Action Subsystem1/MATLAB Function2 ==
  data: index input; y output; value input
function y = fcn(index,value)

y = value(index);

== matlab function case14/Switch Case Action Subsystem1/For Iterator Subsystem/GetGpsL1C/If Action Subsystem/Subsystem/For Iterator Subsystem1/If Action Subsystem2/If Action Subsystem/MATLAB Function ==
  data: Ca_code input; index input; Ca_code output
function Ca_code = fcn(Ca_code,index)
  
   Ca_code(index)=1;
end

== matlab function case14/Switch Case Action Subsystem1/For Iterator Subsystem/GetGpsL1C/If Action Subsystem/Subsystem/For Iterator Subsystem1/If Action Subsystem/If Action Subsystem/MATLAB Function1 ==
  data: value input; y output; index input
function y = fcn(value,index)

y = value(index);

== matlab function case14/Switch Case Action Subsystem2/MATLAB Function ==
  data: ca_code output
function ca_code = fcn()
    ca_code=zeros(1,1023);

== matlab function case14/Switch Case Action Subsystem1/For Iterator Subsystem/GetGpsL1C/If Action Subsystem/Subsystem/For Iterator Subsystem1/If Action Subsystem/If Action Subsystem/MATLAB Function ==
  data: index input; ca_code_14 output; weil_index_p input; ca_code_14 input
function ca_code_14 = fcn(index,weil_index_p, ca_code_14)
    ca_code_14(index)=weil_index_p;

== matlab function case14/Switch Case Action Subsystem1/For Iterator Subsystem/GetGpsL1C/If Action Subsystem/Subsystem/For Iterator Subsystem2/MATLAB Function ==
  data: value input; value output; index input; index1 input
 function value = fcn(value,index,index1)

value(index+index1) = value(index1);

== matlab function case14/Switch Case Action Subsystem1/For Iterator Subsystem/GetGpsL1C/If Action Subsystem/Subsystem/For Iterator Subsystem1/If Action Subsystem/If Action Subsystem1/MATLAB Function1 ==
  data: index input; ca_code_14 output; weil_index_p input; ca_code_14 input
function ca_code_14 = fcn(index,weil_index_p, ca_code_14)
    ca_code_14(index)=weil_index_p;

== matlab function case14/Switch Case Action Subsystem1/For Iterator Subsystem/GetGpsL1C/If Action Subsystem/Subsystem/For Iterator Subsystem/If Action Subsystem/MATLAB Function2 ==
  data: index input; y output; value input
function y = fcn(index,value)

y = value(index);

== matlab function case14/Switch Case Action Subsystem1/For Iterator Subsystem/MATLAB Function3 ==
  data: weil_seq_p output
function weil_seq_p = fcn()
    weil_seq_p=zeros(1,10223);

== matlab function case14/Switch Case Action Subsystem1/For Iterator Subsystem/GetGpsL1C/If Action Subsystem/Subsystem/For Iterator Subsystem/If Action Subsystem1/MATLAB Function3 ==
  data: index input; y output; value input
function y = fcn(index,value)

y = value(index);

== matlab function case14/Switch Case Action Subsystem1/For Iterator Subsystem/GetGpsL1C/If Action Subsystem/Subsystem/For Iterator Subsystem/If Action Subsystem/MATLAB Function1 ==
  data: index input; y output; value input
function y = fcn(index,value)

y = value(index);

== matlab function case14/Switch Case Action Subsystem1/For Iterator Subsystem/GetGpsL1C/If Action Subsystem/Subsystem/For Iterator Subsystem1/If Action Subsystem2/MATLAB Function ==
  data: index_relational input; flag_p_out output; flag_p input; index input
function flag_p_out = fcn(index_relational, flag_p,index)
if index== 10223
    debug=0;
end
       if index_relational==1
          flag_p_out=1;
       else
           flag_p_out=flag_p;
       end

== matlab function case14/Switch Case Action Subsystem3/MATLAB Function ==
  data: ca_code output
function ca_code = fcn()
    ca_code=zeros(1,10244);

== matlab function case14/Switch Case Action Subsystem1/For Iterator Subsystem/MATLAB Function2 ==
  data: value input; y output; index input
function y = fcn(value,index)

y = value(index);

== matlab function case14/Switch Case Action Subsystem1/For Iterator Subsystem/MATLAB Function1 ==
  data: value input; y output; index input
function y = fcn(value,index)

y = value(index);

== matlab function case14/Switch Case Action Subsystem1/For Iterator Subsystem/GetGpsL1C/If Action Subsystem/Subsystem/For Iterator Subsystem1/If Action Subsystem/If Action Subsystem1/MATLAB Function2 ==
  data: weil_seq_p_index input; y output; index input
function y = fcn(weil_seq_p_index, index)
  if index== 10229
    debug=0;
  end
  if index<8
      y=1;
  else
      y=weil_seq_p_index(index-7);
  end

== matlab function case14/Switch Case Action Subsystem1/For Iterator Subsystem/Reverse32bit()/ConvertChar2hex/For Iterator Subsystem/MATLAB Function1 ==
  data: value input; y output; index input
function y = fcn(value,index)

y = value(index);

== matlab function case14/Switch Case Action Subsystem1/For Iterator Subsystem/Reverse32bit()/ConvertChar2hex/For Iterator Subsystem/MATLAB Function2 ==
  data: value input; y output; index input
function y = fcn(value,index)

y = value(index);

== matlab function case14/Switch Case Action Subsystem1/For Iterator Subsystem/Reverse32bit()/ConvertChar2hex/For Iterator Subsystem/MATLAB Function3 ==
  data: value input; y output; index input
function y = fcn(value,index)

y = value(index);

== matlab function case14/Switch Case Action Subsystem1/For Iterator Subsystem/Reverse32bit()/ConvertChar2hex/For Iterator Subsystem/MATLAB Function4 ==
  data: value input; y output; index input
function y = fcn(value,index)

y = value(index);

== matlab function case14/Switch Case Action Subsystem1/For Iterator Subsystem/Reverse32bit()/For Iterator Subsystem/For Iterator Subsystem/MATLAB Function ==
  data: y output
function y = fcn()
        for index=31
            index-- 
        end
y = index;

== matlab function case14/Switch Case Action Subsystem1/For Iterator Subsystem/Reverse32bit()/For Iterator Subsystem/For Iterator Subsystem/MATLAB Function1 ==
  data: value input; y output; index input
function y = fcn(value,index)

y = value(index);

== matlab function case14/Switch Case Action Subsystem1/For Iterator Subsystem/Reverse32bit()/For Iterator Subsystem/For Iterator Subsystem/MATLAB Function2 ==
  data: value input; y output; index input
function y = fcn(value,index)

y = value(index);

== matlab function case14/Switch Case Action Subsystem1/For Iterator Subsystem/GetGpsL1C/If Action Subsystem/Subsystem/For Iterator Subsystem1/If Action Subsystem2/If Action Subsystem2/MATLAB Function ==
  data: u input; y output
function y = fcn(u)
u=int32(1);
y =u;
